simulink subsystem "FORCESANDTORQUES"  (R2025b)
settings: Solver=VariableStepAuto  StartTime=0.0  StopTime=10.0  RelTol=1e-3
model mask{refSurf=0, dc=0, rwAllocationMatrix=0, rwInertias=0, mtqAllocationMatrix=0, rcsPositionMatrix=0, rcsDirectionMatrix=0}
  mask prompts: refSurf "Reference aerodynamic surface [m2]"; dc "Drag coefficient [-]"; rwAllocationMatrix "RW allocation matrix"; rwInertias "Rotational inertia moments [kgm2]"; mtqAllocationMatrix "MTQ allocation matrix"; rcsPositionMatrix "RCS position matrix"; rcsDirectionMatrix "RCS direction matrix"
libraries: aerolibutil x3, matrix_library x2, sharedutil x2
settings Model: Creator=antoniohernandez-rodiciomateos  LastModifiedBy=antoniohernandez-rodiciomateos

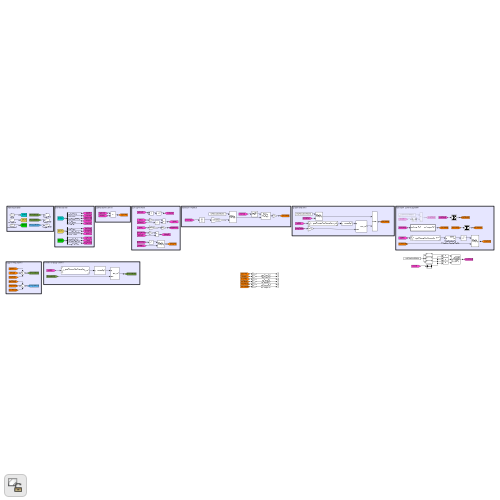
[thumbnail: Simulink's stored preview of the top-level diagram]
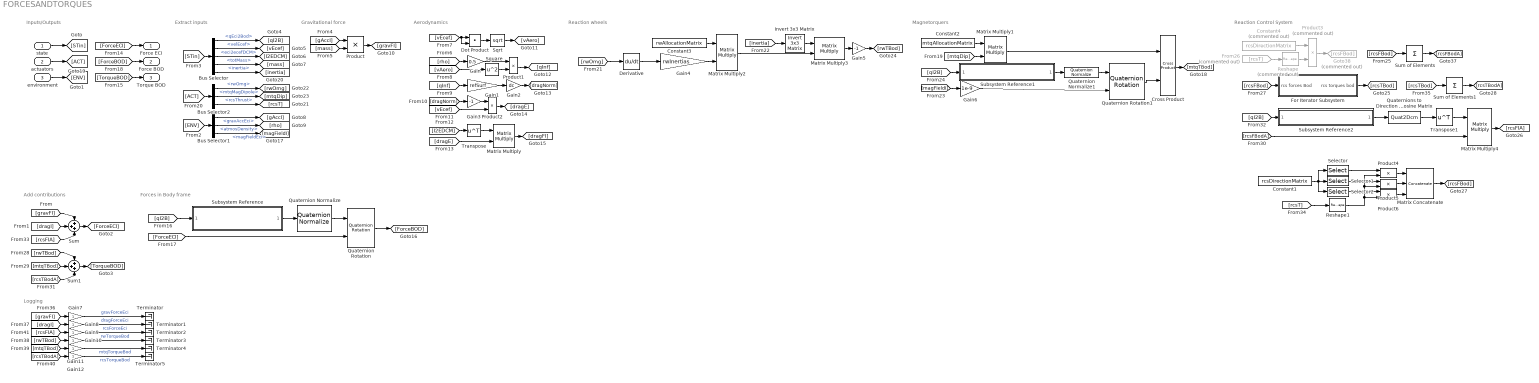
== system FORCESANDTORQUES ==
  note: Inputs/Outputs
  note: Extract inputs
  note: Gravitational force
  note: Aerodynamics
  note: Add contributions
  note: Forces in Body frame
  note: Reaction wheels
  note: Magnetorquers
  note: Reaction Control System
  note: Logging
  state : Inport  OutDataTypeStr=Bus: state_bus
  actuators : Inport  Port=2
  environment : Inport  Port=3  OutDataTypeStr=Bus: environment_bus
  Bus Selector : BusSelector  OutputSignals=qEci2Bod,velEcef,eci2ecefDCM,totMass,inertia
  Bus Selector1 : BusSelector  OutputSignals=gravAccEci,atmosDensity,magFieldEci
  Bus Selector2 : BusSelector  OutputSignals=rwOmg,mtqMagDipole,rcsThrust
  Constant1 : Constant  Value=rcsDirectionMatrix
  Constant2 : Constant  Value=mtqAllocationMatrix
  Constant3 : Constant  Value=rwAllocationMatrix
  Constant4 : Constant  Commented=on  Value=rcsDirectionMatrix
  Cross Product : matrix_library/Cross Product
  Derivative : Derivative
  Dot Product : DotProduct  OutDataTypeStr=Inherit: Inherit via internal rule
  For Iterator Subsystem : Subsystem  TreatAsAtomicUnit=on
  From26 : From  Commented=on  GotoTag=rcsT
  Gain : Gain  Gain=0.5
  Gain1 : Gain  Gain=refSurf
  Gain{7..12} (6 alike) : Gain
  Gain2 : Gain  Gain=dc
  Gain3 : Gain  Gain=-1
  Gain4 : Gain  Gain=rwInertias
  Gain5 : Gain  Gain=-1
  Gain6 : Gain  Gain=1e-9
  Goto38 : Goto  Commented=on  GotoTag=rcsFBod
  Invert 3x3 Matrix : aerolibutil/Invert  3x3 Matrix
  Matrix Concatenate : Concatenate  NumInputs=3  Mode=Multidimensional array
  Matrix Multiply{,1..4} (5 alike) : Product  Multiplication=Matrix(*)
  Product{,1..2,4..6} (6 alike) : Product
  Product3 : Product  Commented=on
  Quaternion Normalize : sharedutil/Quaternion Normalize  aMode=aMode
  Quaternion Normalize1 : sharedutil/Quaternion Normalize  aMode=aMode
  Quaternion Rotation : aerolibutil/Quaternion Rotation
  Quaternion Rotation1 : aerolibutil/Quaternion Rotation
  Quaternions to Direction Cosine Matrix : Quat2Dcm
  Reshape : Reshape  Commented=on  OutputDimensionality=Row vector (2-D)
  Reshape1 : Reshape  OutputDimensionality=Row vector (2-D)
  Selector : Selector  NumberOfDimensions=2  InputPortWidth=3  IndexOptions=Index vector (dialog),Index vector (dialog)  Indices=[1],[1:12]  OutputSizes=1,1
  Selector1 : Selector  NumberOfDimensions=2  InputPortWidth=3  IndexOptions=Index vector (dialog),Index vector (dialog)  Indices=[2],[1:12]  OutputSizes=1,1
  Selector2 : Selector  NumberOfDimensions=2  InputPortWidth=3  IndexOptions=Index vector (dialog),Index vector (dialog)  Indices=[3],[1:12]  OutputSizes=1,1
  Sqrt : Sqrt
  Square : Math  Operator=square
  Subsystem Reference : Subsystem  ReferencedSubsystem=quatConventionConverter  conversion=q4 to q0
  Subsystem Reference1 : Subsystem  ReferencedSubsystem=quatConventionConverter  conversion=q4 to q0
  Subsystem Reference2 : Subsystem  ReferencedSubsystem=quatConventionConverter  conversion=q4 to q0
  Sum : Sum  Inputs=+++
  Sum of Elements : Sum  Inputs=+  CollapseMode=Specified dimension  CollapseDim=2
  Sum of Elements1 : Sum  Inputs=+  CollapseMode=Specified dimension  CollapseDim=2
  Sum1 : Sum  Inputs=+++
  Terminator{,1..5} (6 alike) : Terminator
  Transpose : Math  Operator=transpose
  Transpose1 : Math  Operator=transpose
  Force ECI : Outport  OutDataTypeStr=double  PortDimensions=[3 1]
  Force BOD : Outport  Port=2  OutDataTypeStr=double  PortDimensions=[3 1]
  Torque BOD : Outport  Port=3  OutDataTypeStr=double  PortDimensions=[3 1]
  wires:
  actuators/1 -> [ACT]
  state/1 -> [STin]
  environment/1 -> [ENV]
  [ForceECI] -> Force ECI/1
  [STin] -> Bus Selector/1
  Bus Selector/1 -> [qI2B]  "<qEci2Bod>"
  Bus Selector/2 -> [vEcef]  "<velEcef>"
  Bus Selector/3 -> [I2EDCM]  "<eci2ecefDCM>"
  Bus Selector/4 -> [mass]  "<totMass>"
  [ENV] -> Bus Selector1/1
  Bus Selector1/1 -> [gAccI]  "<gravAccEci>"
  Bus Selector1/2 -> [rho]  "<atmosDensity>"
  [gAccI] -> Product/1
  [mass] -> Product/2
  Product/1 -> [gravFI]
  [vEcef] -> Dot Product/2, Dot Product/1
  Dot Product/1 -> Sqrt/1
  Sqrt/1 -> [vAero]
  [rho] -> Gain/1
  [vAero] -> Square/1
  Gain/1 -> Product1/1
  Square/1 -> Product1/2
  Product1/1 -> [qInf]
  [qInf] -> Gain1/1
  Gain1/1 -> Gain2/1
  Gain2/1 -> [dragNorm]
  [dragNorm] -> Gain3/1
  Gain3/1 -> Product2/1
  [vEcef] -> Product2/2
  Product2/1 -> [dragE]
  [I2EDCM] -> Transpose/1
  Transpose/1 -> Matrix Multiply/1
  [dragE] -> Matrix Multiply/2
  Matrix Multiply/1 -> [dragFI]
  [TorqueBOD] -> Torque BOD/1
  [gravFI] -> Sum/1
  [dragI] -> Sum/2
  Sum/1 -> [ForceECI]
  [qI2B] -> Subsystem Reference/1
  Subsystem Reference/1 -> Quaternion Normalize/1
  Quaternion Normalize/1 -> Quaternion Rotation/1
  [ForceECI] -> Quaternion Rotation/2
  Quaternion Rotation/1 -> [ForceBOD]
  [ForceBOD] -> Force BOD/1
  Bus Selector1/3 -> [magFieldI]  "<magFieldEci>"
  Bus Selector/5 -> [inertia]  "<inertia>"
  [ACT] -> Bus Selector2/1
  Bus Selector2/1 -> [rwOmg]  "<rwOmg>"
  Bus Selector2/2 -> [mtqDip]  "<mtqMagDipole>"
  Bus Selector2/3 -> [rcsT]  "<rcsThrust>"
  [rwOmg] -> Derivative/1
  Derivative/1 -> Gain4/1
  Gain4/1 -> Matrix Multiply2/2
  Constant3/1 -> Matrix Multiply2/1
  Matrix Multiply2/1 -> Matrix Multiply3/2
  [inertia] -> Invert 3x3 Matrix/1
  Invert 3x3 Matrix/1 -> Matrix Multiply3/1
  Constant2/1 -> Matrix Multiply1/1
  [mtqDip] -> Matrix Multiply1/2
  Subsystem Reference1/1 -> Quaternion Normalize1/1
  Quaternion Normalize1/1 -> Quaternion Rotation1/1
  [qI2B] -> Subsystem Reference1/1
  Matrix Multiply1/1 -> Cross Product/1
  Quaternion Rotation1/1 -> Cross Product/2
  Cross Product/1 -> [mtqTBod]
  Constant4/1 -> Product3/1
  From26/1 -> Reshape/1
  Reshape/1 -> Product3/2
  Sum of Elements/1 -> [rcsFBodA]
  Product3/1 -> Goto38/1
  Matrix Multiply3/1 -> Gain5/1
  Gain5/1 -> [rwTBod]
  [rcsFBod] -> Sum of Elements/1
  [rcsFBod] -> For Iterator Subsystem/1(rcs forces Bod)
  For Iterator Subsystem/1(rcs torques bod) -> [rcsTBod]
  [mtqTBod] -> Sum1/2
  Sum1/1 -> [TorqueBOD]
  [rwTBod] -> Sum1/1
  [rcsTBodA] -> Sum1/3
  Subsystem Reference2/1 -> Quaternions to Direction Cosine Matrix/1
  Quaternions to Direction Cosine Matrix/1 -> Transpose1/1
  [qI2B] -> Subsystem Reference2/1
  Transpose1/1 -> Matrix Multiply4/1
  [rcsFBodA] -> Matrix Multiply4/2
  Matrix Multiply4/1 -> [rcsFIA]
  [rcsFIA] -> Sum/3
  Constant1/1 -> Selector1/1, Selector/1, Selector2/1
  Selector/1 -> Product4/1
  Selector1/1 -> Product5/1
  Selector2/1 -> Product6/1
  Product4/1 -> Matrix Concatenate/1
  Product5/1 -> Matrix Concatenate/2
  Product6/1 -> Matrix Concatenate/3
  Matrix Concatenate/1 -> [rcsFBod]
  [rcsT] -> Reshape1/1
  Reshape1/1 -> Product4/2, Product5/2, Product6/2
  [rcsTBod] -> Sum of Elements1/1
  Sum of Elements1/1 -> [rcsTBodA]
  [magFieldI] -> Gain6/1
  Gain6/1 -> Quaternion Rotation1/2
  [gravFI] -> Gain7/1
  [dragI] -> Gain8/1
  [rcsFIA] -> Gain9/1
  [rwTBod] -> Gain10/1
  [mtqTBod] -> Gain11/1
  [rcsTBodA] -> Gain12/1
  Gain7/1 -> Terminator/1  "gravForceEci"
  Gain8/1 -> Terminator1/1  "dragForceEci"
  Gain9/1 -> Terminator2/1  "rcsForceEci"
  Gain10/1 -> Terminator3/1  "rwTorqueBod"
  Gain11/1 -> Terminator4/1  "mtqTorqueBod"
  Gain12/1 -> Terminator5/1  "rcsTorqueBod"

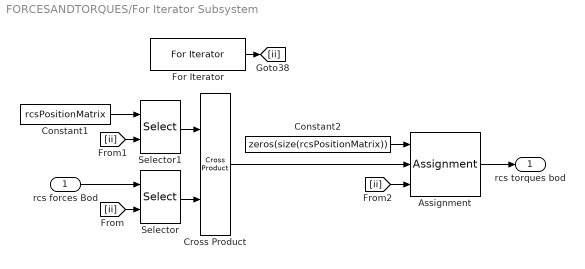
== system FORCESANDTORQUES/For Iterator Subsystem ==
  rcs forces Bod : Inport
  Assignment : Assignment  NumberOfDimensions=2  DiagnosticForDimensions=Warning  IndexOptions=Index vector (dialog),Index vector (port)  Indices=[1 2 3],1  OutputSizes=1,1
  Constant1 : Constant  Value=rcsPositionMatrix
  Constant2 : Constant  Value=zeros(size(rcsPositionMatrix))
  Cross Product : matrix_library/Cross Product
  For Iterator : ForIterator  IterationLimit=size(rcsPositionMatrix, 2)
  Selector : Selector  NumberOfDimensions=2  InputPortWidth=3  IndexOptions=Index vector (dialog),Index vector (port)  Indices=[1 2 3],1  OutputSizes=1,1
  Selector1 : Selector  NumberOfDimensions=2  InputPortWidth=3  IndexOptions=Index vector (dialog),Index vector (port)  Indices=[1 2 3],1  OutputSizes=1,1
  rcs torques bod : Outport
  wires:
  Constant2/1 -> Assignment/1
  [ii] -> Assignment/3
  Assignment/1 -> rcs torques bod/1
  Cross Product/1 -> Assignment/2
  Selector/1 -> Cross Product/2
  Selector1/1 -> Cross Product/1
  [ii] -> Selector1/2
  Constant1/1 -> Selector1/1
  [ii] -> Selector/2
  For Iterator/1 -> [ii]
  rcs forces Bod/1 -> Selector/1
